simulink model "SimulationBOP"  (R2021a)
settings: Solver=VariableStepAuto  StartTime=0.0  StopTime=10.0  RelTol=1e-3
values from neighbouring files (symbols this model uses):
  ds = 0.014    [stepinfo.m]
  g = -9.81    [stepinfo.m]
  Ib = (2/5)*mb*(rb)^2    (= 4.3483784e-06)    [stepinfo.m]
  Lpx = 0.115    [stepinfo.m]
  mb = 0.0674    [stepinfo.m]
  rb = 0.0127    [stepinfo.m]
settings Model: Creator=josef  LastModifiedBy=josef

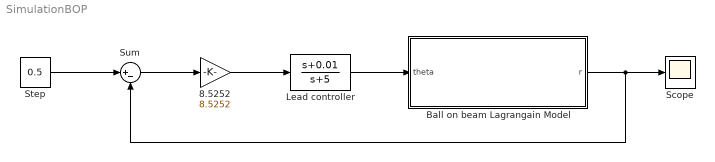
== system SimulationBOP ==
  8.5252 : Gain  Gain=8.5252
  Ball on beam Lagrangain Model : Subsystem
  Lead controller : TransferFcn  Numerator=[1 0.01]  Denominator=[1 5]
  Scope : Scope
  Step : Constant  Value=0.5
  Sum : Sum  Inputs=|+-
  wires:
  Step/1 -> Sum/1
  Sum/1 -> 8.5252/1
  8.5252/1 -> Lead controller/1
  Lead controller/1 -> Ball on beam Lagrangain Model/1(theta)
  Ball on beam Lagrangain Model/1(r) -> Sum/2, Scope/1

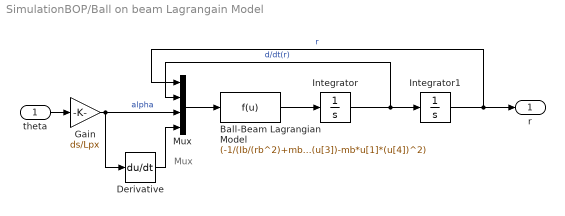
== system SimulationBOP/Ball on beam Lagrangain Model ==
  note: Mux
  theta : Inport
  Ball-Beam Lagrangian Model : Fcn  Expr=(-1/(Ib/(rb^2)+mb))*(mb*g*sin(u[3])-mb*u[1]*(u[4])^2)
  Derivative : Derivative
  Gain : Gain  Gain=ds/Lpx
  Integrator : Integrator
  Integrator1 : Integrator
  Mux : Mux
  r : Outport
  wires:
  Derivative/1 -> Mux/4
  Integrator/1 -> Mux/2, Integrator1/1  "d/dt(r)"
  Integrator1/1 -> Mux/1, r/1  "r"
  theta/1 -> Gain/1
  Gain/1 -> Derivative/1, Mux/3  "alpha"
  Ball-Beam Lagrangian Model/1 -> Integrator/1
  Mux/1 -> Ball-Beam Lagrangian Model/1
